simulink model "sm_import_stewart_platform"  (R2021b)
settings: Solver=ode45  StartTime=0.0  StopTime=10.0  RelTol=1e-3  EnableMultiTasking=on
model workspace (MATLAB code in the model file):
  | % The six origin vectors correspond to the six legs of the Stewart platform
  | stewart_pos_base = [0.0962 0 -0.0336; 0.0772 0 -0.0665;-0.0742 0 -0.0599;...
  |     -0.0962 0 -0.0336; -0.0190 0 0.1001;0.019 0 0.1001];
  | 
  | % Corresponding body points on the top plate
  | stewart_body_pts = [0.0607 0 0.0203; 0.0128 0 -0.0628; -0.0145 0 -0.0669; ...
  |     -0.0652 0 0.0208; -0.0507 0 0.046; 0.0507 0 0.046]';
  | 
  | % Leg length
  | leg_length = 0.19*ones(1,6);
undefined symbols (not defined in the file): X, Y, Z
libraries: sm_lib x1374, nesl_utility x19
(part 17 of 28)

== system sm_import_stewart_platform/Stewart Platform/Imported Stewart Platform/ActuatorAssm1_2/DrivenAssm_1_RIGID/CeramicStrip5010_2_RIGID ==
  ReferenceFrame : sm_lib/Frames and Transforms/Reference Frame
  Solid : sm_lib/Body Elements/File Solid  ExtGeomFileName=CeramicStrip5010_Default_sldprt.STL  UnitType=Custom  ExtGeomFileUnits=cm  StepReaderType=HEX  ExportConvexHullGeometry=off  InertiaType=Custom  Mass=0.0012937499999999978  MassUnits=kg  CenterOfMass=[-0.47402595951185544 0.93613171356507663 0]  CenterOfMassUnits=cm  MomentsOfInertia=[0.006066878906249993 0.0061722656249999933 0.00011023828124999996]  MomentsOfInertiaUnits=kg*cm^2  ProductsOfInertia=[0 0 0]  ProductsOfInertiaUnits=kg*cm^2  BasedOnType=Density  Density=1000  DensityUnits=kg/(m^3)  DoExposeReferenceFrame=on  SerializedFrames=<Frames/>  GraphicType=FromGeometry  MarkerShape=Sphere  MarkerSize=10  MarkerSizeUnits=m  GraphicVisPropType=SimpleVisualProperties  GraphicDiffuseColor=[0.95999999999999996 0.95999999999999996 0.95999999999999996]  GraphicSpecularColor=[0.5 0.5 0.5 1.0]  GraphicAmbientColor=[0.15 0.15 0.15 1.0]  GraphicEmissiveColor=[0.0 0.0 0.0 1.0]  GraphicShininess=75  GraphicOpacity=1
  F : PMIOPort  Side=Left
  connections:
  ReferenceFrame/RConn1 -- Solid/RConn1 -- F/RConn1

== system sm_import_stewart_platform/Stewart Platform/Imported Stewart Platform/ActuatorAssm1_2/DrivenAssm_1_RIGID/GratingStrip5010_1_RIGID ==
  ReferenceFrame : sm_lib/Frames and Transforms/Reference Frame
  Solid : sm_lib/Body Elements/File Solid  ExtGeomFileName=GratingStrip5010_Default_sldprt.STL  UnitType=Custom  ExtGeomFileUnits=cm  StepReaderType=HEX  ExportConvexHullGeometry=off  InertiaType=Custom  Mass=0.00056172468299999889  MassUnits=kg  CenterOfMass=[-0.84754852632874456 1.2395216473722859 3.0000000000000004]  CenterOfMassUnits=cm  MomentsOfInertia=[0.001685186808580852 0.0017040491686085529 1.8887879189411595e-05]  MomentsOfInertiaUnits=kg*cm^2  ProductsOfInertia=[0 0 0]  ProductsOfInertiaUnits=kg*cm^2  BasedOnType=Density  Density=1000  DensityUnits=kg/(m^3)  DoExposeReferenceFrame=on  SerializedFrames=<Frames/>  GraphicType=FromGeometry  MarkerShape=Sphere  MarkerSize=10  MarkerSizeUnits=m  GraphicVisPropType=SimpleVisualProperties  GraphicDiffuseColor=[0.71905882352941175 0.57976470588235285 0.21835294117647058]  GraphicSpecularColor=[0.5 0.5 0.5 1.0]  GraphicAmbientColor=[0.15 0.15 0.15 1.0]  GraphicEmissiveColor=[0.0 0.0 0.0 1.0]  GraphicShininess=75  GraphicOpacity=1
  F : PMIOPort  Side=Left
  connections:
  ReferenceFrame/RConn1 -- Solid/RConn1 -- F/RConn1

== system sm_import_stewart_platform/Stewart Platform/Imported Stewart Platform/ActuatorAssm1_2/DrivenAssm_1_RIGID/Recessed_Pan_Head_Screw_M2x8_48_Z_10_RIGID ==
  ReferenceFrame : sm_lib/Frames and Transforms/Reference Frame
  Solid : sm_lib/Body Elements/File Solid  ExtGeomFileName=Recessed_Pan_Head_Screw_M2x8_48_Z_Default_sldprt.STL  UnitType=Custom  ExtGeomFileUnits=cm  StepReaderType=HEX  ExportConvexHullGeometry=off  InertiaType=Custom  Mass=0.00030420054001085506  MassUnits=kg  CenterOfMass=[0.23057963245570592 -4.2158298307861626e-10 -1.6472469656016965e-11]  CenterOfMassUnits=cm  MomentsOfInertia=[3.0541038740142581e-06 2.6916548970402947e-05 2.6916548962268568e-05]  MomentsOfInertiaUnits=kg*cm^2  ProductsOfInertia=[0 0 0]  ProductsOfInertiaUnits=kg*cm^2  BasedOnType=Density  Density=1000  DensityUnits=kg/(m^3)  DoExposeReferenceFrame=on  SerializedFrames=<Frames/>  GraphicType=FromGeometry  MarkerShape=Sphere  MarkerSize=10  MarkerSizeUnits=m  GraphicVisPropType=SimpleVisualProperties  GraphicDiffuseColor=[0.72282352941176464 0.72282352941176464 0.72282352941176464]  GraphicSpecularColor=[0.5 0.5 0.5 1.0]  GraphicAmbientColor=[0.15 0.15 0.15 1.0]  GraphicEmissiveColor=[0.0 0.0 0.0 1.0]  GraphicShininess=75  GraphicOpacity=1
  F : PMIOPort  Side=Left
  connections:
  ReferenceFrame/RConn1 -- Solid/RConn1 -- F/RConn1

== system sm_import_stewart_platform/Stewart Platform/Imported Stewart Platform/ActuatorAssm1_2/DrivenAssm_1_RIGID/Recessed_Pan_Head_Screw_M2x8_48_Z_1_RIGID ==
  ReferenceFrame : sm_lib/Frames and Transforms/Reference Frame
  Solid : sm_lib/Body Elements/File Solid  ExtGeomFileName=Recessed_Pan_Head_Screw_M2x8_48_Z_Default_sldprt.STL  UnitType=Custom  ExtGeomFileUnits=cm  StepReaderType=HEX  ExportConvexHullGeometry=off  InertiaType=Custom  Mass=0.00030420054001085506  MassUnits=kg  CenterOfMass=[0.23057963245570592 -4.2158298307861626e-10 -1.6472469656016965e-11]  CenterOfMassUnits=cm  MomentsOfInertia=[3.0541038740142581e-06 2.6916548970402947e-05 2.6916548962268568e-05]  MomentsOfInertiaUnits=kg*cm^2  ProductsOfInertia=[0 0 0]  ProductsOfInertiaUnits=kg*cm^2  BasedOnType=Density  Density=1000  DensityUnits=kg/(m^3)  DoExposeReferenceFrame=on  SerializedFrames=<Frames/>  GraphicType=FromGeometry  MarkerShape=Sphere  MarkerSize=10  MarkerSizeUnits=m  GraphicVisPropType=SimpleVisualProperties  GraphicDiffuseColor=[0.72282352941176464 0.72282352941176464 0.72282352941176464]  GraphicSpecularColor=[0.5 0.5 0.5 1.0]  GraphicAmbientColor=[0.15 0.15 0.15 1.0]  GraphicEmissiveColor=[0.0 0.0 0.0 1.0]  GraphicShininess=75  GraphicOpacity=1
  F : PMIOPort  Side=Left
  connections:
  ReferenceFrame/RConn1 -- Solid/RConn1 -- F/RConn1

== system sm_import_stewart_platform/Stewart Platform/Imported Stewart Platform/ActuatorAssm1_2/DrivenAssm_1_RIGID/Recessed_Pan_Head_Screw_M2x8_48_Z_2_RIGID ==
  ReferenceFrame : sm_lib/Frames and Transforms/Reference Frame
  Solid : sm_lib/Body Elements/File Solid  ExtGeomFileName=Recessed_Pan_Head_Screw_M2x8_48_Z_Default_sldprt.STL  UnitType=Custom  ExtGeomFileUnits=cm  StepReaderType=HEX  ExportConvexHullGeometry=off  InertiaType=Custom  Mass=0.00030420054001085506  MassUnits=kg  CenterOfMass=[0.23057963245570592 -4.2158298307861626e-10 -1.6472469656016965e-11]  CenterOfMassUnits=cm  MomentsOfInertia=[3.0541038740142581e-06 2.6916548970402947e-05 2.6916548962268568e-05]  MomentsOfInertiaUnits=kg*cm^2  ProductsOfInertia=[0 0 0]  ProductsOfInertiaUnits=kg*cm^2  BasedOnType=Density  Density=1000  DensityUnits=kg/(m^3)  DoExposeReferenceFrame=on  SerializedFrames=<Frames/>  GraphicType=FromGeometry  MarkerShape=Sphere  MarkerSize=10  MarkerSizeUnits=m  GraphicVisPropType=SimpleVisualProperties  GraphicDiffuseColor=[0.72282352941176464 0.72282352941176464 0.72282352941176464]  GraphicSpecularColor=[0.5 0.5 0.5 1.0]  GraphicAmbientColor=[0.15 0.15 0.15 1.0]  GraphicEmissiveColor=[0.0 0.0 0.0 1.0]  GraphicShininess=75  GraphicOpacity=1
  F : PMIOPort  Side=Left
  connections:
  ReferenceFrame/RConn1 -- Solid/RConn1 -- F/RConn1

== system sm_import_stewart_platform/Stewart Platform/Imported Stewart Platform/ActuatorAssm1_2/DrivenAssm_1_RIGID/Recessed_Pan_Head_Screw_M2x8_48_Z_3_RIGID ==
  ReferenceFrame : sm_lib/Frames and Transforms/Reference Frame
  Solid : sm_lib/Body Elements/File Solid  ExtGeomFileName=Recessed_Pan_Head_Screw_M2x8_48_Z_Default_sldprt.STL  UnitType=Custom  ExtGeomFileUnits=cm  StepReaderType=HEX  ExportConvexHullGeometry=off  InertiaType=Custom  Mass=0.00030420054001085506  MassUnits=kg  CenterOfMass=[0.23057963245570592 -4.2158298307861626e-10 -1.6472469656016965e-11]  CenterOfMassUnits=cm  MomentsOfInertia=[3.0541038740142581e-06 2.6916548970402947e-05 2.6916548962268568e-05]  MomentsOfInertiaUnits=kg*cm^2  ProductsOfInertia=[0 0 0]  ProductsOfInertiaUnits=kg*cm^2  BasedOnType=Density  Density=1000  DensityUnits=kg/(m^3)  DoExposeReferenceFrame=on  SerializedFrames=<Frames/>  GraphicType=FromGeometry  MarkerShape=Sphere  MarkerSize=10  MarkerSizeUnits=m  GraphicVisPropType=SimpleVisualProperties  GraphicDiffuseColor=[0.72282352941176464 0.72282352941176464 0.72282352941176464]  GraphicSpecularColor=[0.5 0.5 0.5 1.0]  GraphicAmbientColor=[0.15 0.15 0.15 1.0]  GraphicEmissiveColor=[0.0 0.0 0.0 1.0]  GraphicShininess=75  GraphicOpacity=1
  F : PMIOPort  Side=Left
  connections:
  ReferenceFrame/RConn1 -- Solid/RConn1 -- F/RConn1

== system sm_import_stewart_platform/Stewart Platform/Imported Stewart Platform/ActuatorAssm1_2/DrivenAssm_1_RIGID/Recessed_Pan_Head_Screw_M2x8_48_Z_4_RIGID ==
  ReferenceFrame : sm_lib/Frames and Transforms/Reference Frame
  Solid : sm_lib/Body Elements/File Solid  ExtGeomFileName=Recessed_Pan_Head_Screw_M2x8_48_Z_Default_sldprt.STL  UnitType=Custom  ExtGeomFileUnits=cm  StepReaderType=HEX  ExportConvexHullGeometry=off  InertiaType=Custom  Mass=0.00030420054001085506  MassUnits=kg  CenterOfMass=[0.23057963245570592 -4.2158298307861626e-10 -1.6472469656016965e-11]  CenterOfMassUnits=cm  MomentsOfInertia=[3.0541038740142581e-06 2.6916548970402947e-05 2.6916548962268568e-05]  MomentsOfInertiaUnits=kg*cm^2  ProductsOfInertia=[0 0 0]  ProductsOfInertiaUnits=kg*cm^2  BasedOnType=Density  Density=1000  DensityUnits=kg/(m^3)  DoExposeReferenceFrame=on  SerializedFrames=<Frames/>  GraphicType=FromGeometry  MarkerShape=Sphere  MarkerSize=10  MarkerSizeUnits=m  GraphicVisPropType=SimpleVisualProperties  GraphicDiffuseColor=[0.72282352941176464 0.72282352941176464 0.72282352941176464]  GraphicSpecularColor=[0.5 0.5 0.5 1.0]  GraphicAmbientColor=[0.15 0.15 0.15 1.0]  GraphicEmissiveColor=[0.0 0.0 0.0 1.0]  GraphicShininess=75  GraphicOpacity=1
  F : PMIOPort  Side=Left
  connections:
  ReferenceFrame/RConn1 -- Solid/RConn1 -- F/RConn1

== system sm_import_stewart_platform/Stewart Platform/Imported Stewart Platform/ActuatorAssm1_2/DrivenAssm_1_RIGID/Recessed_Pan_Head_Screw_M2x8_48_Z_5_RIGID ==
  ReferenceFrame : sm_lib/Frames and Transforms/Reference Frame
  Solid : sm_lib/Body Elements/File Solid  ExtGeomFileName=Recessed_Pan_Head_Screw_M2x8_48_Z_Default_sldprt.STL  UnitType=Custom  ExtGeomFileUnits=cm  StepReaderType=HEX  ExportConvexHullGeometry=off  InertiaType=Custom  Mass=0.00030420054001085506  MassUnits=kg  CenterOfMass=[0.23057963245570592 -4.2158298307861626e-10 -1.6472469656016965e-11]  CenterOfMassUnits=cm  MomentsOfInertia=[3.0541038740142581e-06 2.6916548970402947e-05 2.6916548962268568e-05]  MomentsOfInertiaUnits=kg*cm^2  ProductsOfInertia=[0 0 0]  ProductsOfInertiaUnits=kg*cm^2  BasedOnType=Density  Density=1000  DensityUnits=kg/(m^3)  DoExposeReferenceFrame=on  SerializedFrames=<Frames/>  GraphicType=FromGeometry  MarkerShape=Sphere  MarkerSize=10  MarkerSizeUnits=m  GraphicVisPropType=SimpleVisualProperties  GraphicDiffuseColor=[0.72282352941176464 0.72282352941176464 0.72282352941176464]  GraphicSpecularColor=[0.5 0.5 0.5 1.0]  GraphicAmbientColor=[0.15 0.15 0.15 1.0]  GraphicEmissiveColor=[0.0 0.0 0.0 1.0]  GraphicShininess=75  GraphicOpacity=1
  F : PMIOPort  Side=Left
  connections:
  ReferenceFrame/RConn1 -- Solid/RConn1 -- F/RConn1

== system sm_import_stewart_platform/Stewart Platform/Imported Stewart Platform/ActuatorAssm1_2/DrivenAssm_1_RIGID/Recessed_Pan_Head_Screw_M2x8_48_Z_6_RIGID ==
  ReferenceFrame : sm_lib/Frames and Transforms/Reference Frame
  Solid : sm_lib/Body Elements/File Solid  ExtGeomFileName=Recessed_Pan_Head_Screw_M2x8_48_Z_Default_sldprt.STL  UnitType=Custom  ExtGeomFileUnits=cm  StepReaderType=HEX  ExportConvexHullGeometry=off  InertiaType=Custom  Mass=0.00030420054001085506  MassUnits=kg  CenterOfMass=[0.23057963245570592 -4.2158298307861626e-10 -1.6472469656016965e-11]  CenterOfMassUnits=cm  MomentsOfInertia=[3.0541038740142581e-06 2.6916548970402947e-05 2.6916548962268568e-05]  MomentsOfInertiaUnits=kg*cm^2  ProductsOfInertia=[0 0 0]  ProductsOfInertiaUnits=kg*cm^2  BasedOnType=Density  Density=1000  DensityUnits=kg/(m^3)  DoExposeReferenceFrame=on  SerializedFrames=<Frames/>  GraphicType=FromGeometry  MarkerShape=Sphere  MarkerSize=10  MarkerSizeUnits=m  GraphicVisPropType=SimpleVisualProperties  GraphicDiffuseColor=[0.72282352941176464 0.72282352941176464 0.72282352941176464]  GraphicSpecularColor=[0.5 0.5 0.5 1.0]  GraphicAmbientColor=[0.15 0.15 0.15 1.0]  GraphicEmissiveColor=[0.0 0.0 0.0 1.0]  GraphicShininess=75  GraphicOpacity=1
  F : PMIOPort  Side=Left
  connections:
  ReferenceFrame/RConn1 -- Solid/RConn1 -- F/RConn1

== system sm_import_stewart_platform/Stewart Platform/Imported Stewart Platform/ActuatorAssm1_2/DrivenAssm_1_RIGID/Recessed_Pan_Head_Screw_M2x8_48_Z_7_RIGID ==
  ReferenceFrame : sm_lib/Frames and Transforms/Reference Frame
  Solid : sm_lib/Body Elements/File Solid  ExtGeomFileName=Recessed_Pan_Head_Screw_M2x8_48_Z_Default_sldprt.STL  UnitType=Custom  ExtGeomFileUnits=cm  StepReaderType=HEX  ExportConvexHullGeometry=off  InertiaType=Custom  Mass=0.00030420054001085506  MassUnits=kg  CenterOfMass=[0.23057963245570592 -4.2158298307861626e-10 -1.6472469656016965e-11]  CenterOfMassUnits=cm  MomentsOfInertia=[3.0541038740142581e-06 2.6916548970402947e-05 2.6916548962268568e-05]  MomentsOfInertiaUnits=kg*cm^2  ProductsOfInertia=[0 0 0]  ProductsOfInertiaUnits=kg*cm^2  BasedOnType=Density  Density=1000  DensityUnits=kg/(m^3)  DoExposeReferenceFrame=on  SerializedFrames=<Frames/>  GraphicType=FromGeometry  MarkerShape=Sphere  MarkerSize=10  MarkerSizeUnits=m  GraphicVisPropType=SimpleVisualProperties  GraphicDiffuseColor=[0.72282352941176464 0.72282352941176464 0.72282352941176464]  GraphicSpecularColor=[0.5 0.5 0.5 1.0]  GraphicAmbientColor=[0.15 0.15 0.15 1.0]  GraphicEmissiveColor=[0.0 0.0 0.0 1.0]  GraphicShininess=75  GraphicOpacity=1
  F : PMIOPort  Side=Left
  connections:
  ReferenceFrame/RConn1 -- Solid/RConn1 -- F/RConn1

== system sm_import_stewart_platform/Stewart Platform/Imported Stewart Platform/ActuatorAssm1_2/DrivenAssm_1_RIGID/Recessed_Pan_Head_Screw_M2x8_48_Z_8_RIGID ==
  ReferenceFrame : sm_lib/Frames and Transforms/Reference Frame
  Solid : sm_lib/Body Elements/File Solid  ExtGeomFileName=Recessed_Pan_Head_Screw_M2x8_48_Z_Default_sldprt.STL  UnitType=Custom  ExtGeomFileUnits=cm  StepReaderType=HEX  ExportConvexHullGeometry=off  InertiaType=Custom  Mass=0.00030420054001085506  MassUnits=kg  CenterOfMass=[0.23057963245570592 -4.2158298307861626e-10 -1.6472469656016965e-11]  CenterOfMassUnits=cm  MomentsOfInertia=[3.0541038740142581e-06 2.6916548970402947e-05 2.6916548962268568e-05]  MomentsOfInertiaUnits=kg*cm^2  ProductsOfInertia=[0 0 0]  ProductsOfInertiaUnits=kg*cm^2  BasedOnType=Density  Density=1000  DensityUnits=kg/(m^3)  DoExposeReferenceFrame=on  SerializedFrames=<Frames/>  GraphicType=FromGeometry  MarkerShape=Sphere  MarkerSize=10  MarkerSizeUnits=m  GraphicVisPropType=SimpleVisualProperties  GraphicDiffuseColor=[0.72282352941176464 0.72282352941176464 0.72282352941176464]  GraphicSpecularColor=[0.5 0.5 0.5 1.0]  GraphicAmbientColor=[0.15 0.15 0.15 1.0]  GraphicEmissiveColor=[0.0 0.0 0.0 1.0]  GraphicShininess=75  GraphicOpacity=1
  F : PMIOPort  Side=Left
  connections:
  ReferenceFrame/RConn1 -- Solid/RConn1 -- F/RConn1

== system sm_import_stewart_platform/Stewart Platform/Imported Stewart Platform/ActuatorAssm1_2/DrivenAssm_1_RIGID/Recessed_Pan_Head_Screw_M2x8_48_Z_9_RIGID ==
  ReferenceFrame : sm_lib/Frames and Transforms/Reference Frame
  Solid : sm_lib/Body Elements/File Solid  ExtGeomFileName=Recessed_Pan_Head_Screw_M2x8_48_Z_Default_sldprt.STL  UnitType=Custom  ExtGeomFileUnits=cm  StepReaderType=HEX  ExportConvexHullGeometry=off  InertiaType=Custom  Mass=0.00030420054001085506  MassUnits=kg  CenterOfMass=[0.23057963245570592 -4.2158298307861626e-10 -1.6472469656016965e-11]  CenterOfMassUnits=cm  MomentsOfInertia=[3.0541038740142581e-06 2.6916548970402947e-05 2.6916548962268568e-05]  MomentsOfInertiaUnits=kg*cm^2  ProductsOfInertia=[0 0 0]  ProductsOfInertiaUnits=kg*cm^2  BasedOnType=Density  Density=1000  DensityUnits=kg/(m^3)  DoExposeReferenceFrame=on  SerializedFrames=<Frames/>  GraphicType=FromGeometry  MarkerShape=Sphere  MarkerSize=10  MarkerSizeUnits=m  GraphicVisPropType=SimpleVisualProperties  GraphicDiffuseColor=[0.72282352941176464 0.72282352941176464 0.72282352941176464]  GraphicSpecularColor=[0.5 0.5 0.5 1.0]  GraphicAmbientColor=[0.15 0.15 0.15 1.0]  GraphicEmissiveColor=[0.0 0.0 0.0 1.0]  GraphicShininess=75  GraphicOpacity=1
  F : PMIOPort  Side=Left
  connections:
  ReferenceFrame/RConn1 -- Solid/RConn1 -- F/RConn1

== system sm_import_stewart_platform/Stewart Platform/Imported Stewart Platform/ActuatorAssm1_2/DrivenAssm_1_RIGID/SV2075_1_RIGID ==
  ReferenceFrame : sm_lib/Frames and Transforms/Reference Frame
  Solid : sm_lib/Body Elements/File Solid  ExtGeomFileName=SV2075_Default_sldprt.STL  UnitType=Custom  ExtGeomFileUnits=cm  StepReaderType=HEX  ExportConvexHullGeometry=off  InertiaType=Custom  Mass=0.0058459106101348196  MassUnits=kg  CenterOfMass=[-0.3298949175327261 0.0096923486215533452 3.75]  CenterOfMassUnits=cm  MomentsOfInertia=[0.027698839272727555 0.027673933267832958 0.00032822959311509738]  MomentsOfInertiaUnits=kg*cm^2  ProductsOfInertia=[0 0 1.1416492577499715e-06]  ProductsOfInertiaUnits=kg*cm^2  BasedOnType=Density  Density=1000  DensityUnits=kg/(m^3)  DoExposeReferenceFrame=on  SerializedFrames=<Frames/>  GraphicType=FromGeometry  MarkerShape=Sphere  MarkerSize=10  MarkerSizeUnits=m  GraphicVisPropType=SimpleVisualProperties  GraphicDiffuseColor=[0.97999999999999998 0.97999999999999998 0.97999999999999998]  GraphicSpecularColor=[0.5 0.5 0.5 1.0]  GraphicAmbientColor=[0.15 0.15 0.15 1.0]  GraphicEmissiveColor=[0.0 0.0 0.0 1.0]  GraphicShininess=75  GraphicOpacity=1
  F : PMIOPort  Side=Left
  connections:
  ReferenceFrame/RConn1 -- Solid/RConn1 -- F/RConn1

== system sm_import_stewart_platform/Stewart Platform/Imported Stewart Platform/ActuatorAssm1_2/DrivenAssm_1_RIGID/SV2075_2_RIGID ==
  ReferenceFrame : sm_lib/Frames and Transforms/Reference Frame
  Solid : sm_lib/Body Elements/File Solid  ExtGeomFileName=SV2075_Default_sldprt.STL  UnitType=Custom  ExtGeomFileUnits=cm  StepReaderType=HEX  ExportConvexHullGeometry=off  InertiaType=Custom  Mass=0.0058459106101348196  MassUnits=kg  CenterOfMass=[-0.3298949175327261 0.0096923486215533452 3.75]  CenterOfMassUnits=cm  MomentsOfInertia=[0.027698839272727555 0.027673933267832958 0.00032822959311509738]  MomentsOfInertiaUnits=kg*cm^2  ProductsOfInertia=[0 0 1.1416492577499715e-06]  ProductsOfInertiaUnits=kg*cm^2  BasedOnType=Density  Density=1000  DensityUnits=kg/(m^3)  DoExposeReferenceFrame=on  SerializedFrames=<Frames/>  GraphicType=FromGeometry  MarkerShape=Sphere  MarkerSize=10  MarkerSizeUnits=m  GraphicVisPropType=SimpleVisualProperties  GraphicDiffuseColor=[0.97999999999999998 0.97999999999999998 0.97999999999999998]  GraphicSpecularColor=[0.5 0.5 0.5 1.0]  GraphicAmbientColor=[0.15 0.15 0.15 1.0]  GraphicEmissiveColor=[0.0 0.0 0.0 1.0]  GraphicShininess=75  GraphicOpacity=1
  F : PMIOPort  Side=Left
  connections:
  ReferenceFrame/RConn1 -- Solid/RConn1 -- F/RConn1

== system sm_import_stewart_platform/Stewart Platform/Imported Stewart Platform/ActuatorAssm1_2/DrivenAssm_1_RIGID/Yoke_1_RIGID ==
  ReferenceFrame : sm_lib/Frames and Transforms/Reference Frame
  Solid : sm_lib/Body Elements/File Solid  ExtGeomFileName=Yoke_Default_sldprt.STL  UnitType=Custom  ExtGeomFileUnits=m  StepReaderType=HEX  ExportConvexHullGeometry=off  InertiaType=Custom  Mass=0.0085668068985893069  MassUnits=kg  CenterOfMass=[3.3036113322449594e-09 4.5392080360257641e-09 0.013809135161090778]  CenterOfMassUnits=m  MomentsOfInertia=[3.6198630707133227e-07 3.7260728672028368e-07 1.1777278033424778e-07]  MomentsOfInertiaUnits=kg*m^2  ProductsOfInertia=[1.5891854780888145e-13 3.9281797530062808e-13 -1.9646780999777998e-13]  ProductsOfInertiaUnits=kg*m^2  BasedOnType=Density  Density=1000  DensityUnits=kg/(m^3)  DoExposeReferenceFrame=on  SerializedFrames=<Frames/>  GraphicType=FromGeometry  MarkerShape=Sphere  MarkerSize=10  MarkerSizeUnits=m  GraphicVisPropType=SimpleVisualProperties  GraphicDiffuseColor=[0.77647058823529413 0.75686274509803919 0.73725490196078436]  GraphicSpecularColor=[0.5 0.5 0.5 1.0]  GraphicAmbientColor=[0.15 0.15 0.15 1.0]  GraphicEmissiveColor=[0.0 0.0 0.0 1.0]  GraphicShininess=75  GraphicOpacity=1
  F : PMIOPort  Side=Left
  connections:
  ReferenceFrame/RConn1 -- Solid/RConn1 -- F/RConn1

== system sm_import_stewart_platform/Stewart Platform/Imported Stewart Platform/ActuatorAssm1_2/DrivenAssm_1_RIGID/pin2_1_RIGID ==
  ReferenceFrame : sm_lib/Frames and Transforms/Reference Frame
  Solid : sm_lib/Body Elements/File Solid  ExtGeomFileName=pin2_Default_sldprt.STL  UnitType=Custom  ExtGeomFileUnits=cm  StepReaderType=HEX  ExportConvexHullGeometry=off  InertiaType=Custom  Mass=0.0030640524011317904  MassUnits=kg  CenterOfMass=[0.62878050766606708 1.2281931362555856e-05 9.2878917417835236e-08]  CenterOfMassUnits=cm  MomentsOfInertia=[0.00015143303511498066 0.00047164024915314555 0.00047162614442519934]  MomentsOfInertiaUnits=kg*cm^2  ProductsOfInertia=[-9.4727819805528836e-10 1.4280711810645117e-10 1.8883664164919476e-08]  ProductsOfInertiaUnits=kg*cm^2  BasedOnType=Density  Density=1000  DensityUnits=kg/(m^3)  DoExposeReferenceFrame=on  SerializedFrames=<Frames/>  GraphicType=FromGeometry  MarkerShape=Sphere  MarkerSize=10  MarkerSizeUnits=m  GraphicVisPropType=SimpleVisualProperties  GraphicDiffuseColor=[0.72282352941176464 0.72282352941176464 0.72282352941176464]  GraphicSpecularColor=[0.5 0.5 0.5 1.0]  GraphicAmbientColor=[0.15 0.15 0.15 1.0]  GraphicEmissiveColor=[0.0 0.0 0.0 1.0]  GraphicShininess=75  GraphicOpacity=1
  F : PMIOPort  Side=Left
  connections:
  ReferenceFrame/RConn1 -- Solid/RConn1 -- F/RConn1

== system sm_import_stewart_platform/Stewart Platform/Imported Stewart Platform/ActuatorAssm2_2/CarrierAssm_1_RIGID/Carrier_Block_1_RIGID ==
  ReferenceFrame : sm_lib/Frames and Transforms/Reference Frame
  Solid : sm_lib/Body Elements/File Solid  ExtGeomFileName=Carrier_Block_Default_sldprt.STL  UnitType=Custom  ExtGeomFileUnits=m  StepReaderType=HEX  ExportConvexHullGeometry=off  InertiaType=Custom  Mass=0.29755503214781071  MassUnits=kg  CenterOfMass=[0.052371592454755117 -0.00023155972844887416 0.0090326123177344834]  CenterOfMassUnits=m  MomentsOfInertia=[0.00011632507036741897 0.00038061460758238494 0.00046776142289895373]  MomentsOfInertiaUnits=kg*m^2  ProductsOfInertia=[-7.7054025601460358e-07 -8.2627224851298449e-06 -5.2656093991147314e-07]  ProductsOfInertiaUnits=kg*m^2  BasedOnType=Density  Density=1000  DensityUnits=kg/(m^3)  DoExposeReferenceFrame=on  SerializedFrames=<Frames/>  GraphicType=FromGeometry  MarkerShape=Sphere  MarkerSize=10  MarkerSizeUnits=m  GraphicVisPropType=SimpleVisualProperties  GraphicDiffuseColor=[0.21568627450980393 0.60784313725490191 1]  GraphicSpecularColor=[0.5 0.5 0.5 1.0]  GraphicAmbientColor=[0.15 0.15 0.15 1.0]  GraphicEmissiveColor=[0.0 0.0 0.0 1.0]  GraphicShininess=75  GraphicOpacity=1
  F : PMIOPort  Side=Left
  connections:
  ReferenceFrame/RConn1 -- Solid/RConn1 -- F/RConn1

== system sm_import_stewart_platform/Stewart Platform/Imported Stewart Platform/ActuatorAssm2_2/CarrierAssm_1_RIGID/Cylinder_Head_Cap_Screw_M3x8_1_RIGID ==
  ReferenceFrame : sm_lib/Frames and Transforms/Reference Frame
  Solid : sm_lib/Body Elements/File Solid  ExtGeomFileName=Cylinder_Head_Cap_Screw_M3x8_Default_sldprt.STL  UnitType=Custom  ExtGeomFileUnits=cm  StepReaderType=HEX  ExportConvexHullGeometry=off  InertiaType=Custom  Mass=0.00075681554585630491  MassUnits=kg  CenterOfMass=[0.18814854043794096 4.2404888903707961e-05 3.0314199022387744e-07]  CenterOfMassUnits=cm  MomentsOfInertia=[1.8441866345461375e-05 7.8616006686727758e-05 7.8603749633107087e-05]  MomentsOfInertiaUnits=kg*cm^2  ProductsOfInertia=[-8.295565631821646e-10 6.6108014175054549e-11 9.2474917315283758e-09]  ProductsOfInertiaUnits=kg*cm^2  BasedOnType=Density  Density=1000  DensityUnits=kg/(m^3)  DoExposeReferenceFrame=on  SerializedFrames=<Frames/>  GraphicType=FromGeometry  MarkerShape=Sphere  MarkerSize=10  MarkerSizeUnits=m  GraphicVisPropType=SimpleVisualProperties  GraphicDiffuseColor=[0.72282352941176464 0.72282352941176464 0.72282352941176464]  GraphicSpecularColor=[0.5 0.5 0.5 1.0]  GraphicAmbientColor=[0.15 0.15 0.15 1.0]  GraphicEmissiveColor=[0.0 0.0 0.0 1.0]  GraphicShininess=75  GraphicOpacity=1
  F : PMIOPort  Side=Left
  connections:
  ReferenceFrame/RConn1 -- Solid/RConn1 -- F/RConn1

== system sm_import_stewart_platform/Stewart Platform/Imported Stewart Platform/ActuatorAssm2_2/CarrierAssm_1_RIGID/Cylinder_Head_Cap_Screw_M3x8_2_RIGID ==
  ReferenceFrame : sm_lib/Frames and Transforms/Reference Frame
  Solid : sm_lib/Body Elements/File Solid  ExtGeomFileName=Cylinder_Head_Cap_Screw_M3x8_Default_sldprt.STL  UnitType=Custom  ExtGeomFileUnits=cm  StepReaderType=HEX  ExportConvexHullGeometry=off  InertiaType=Custom  Mass=0.00075681554585630491  MassUnits=kg  CenterOfMass=[0.18814854043794096 4.2404888903707961e-05 3.0314199022387744e-07]  CenterOfMassUnits=cm  MomentsOfInertia=[1.8441866345461375e-05 7.8616006686727758e-05 7.8603749633107087e-05]  MomentsOfInertiaUnits=kg*cm^2  ProductsOfInertia=[-8.295565631821646e-10 6.6108014175054549e-11 9.2474917315283758e-09]  ProductsOfInertiaUnits=kg*cm^2  BasedOnType=Density  Density=1000  DensityUnits=kg/(m^3)  DoExposeReferenceFrame=on  SerializedFrames=<Frames/>  GraphicType=FromGeometry  MarkerShape=Sphere  MarkerSize=10  MarkerSizeUnits=m  GraphicVisPropType=SimpleVisualProperties  GraphicDiffuseColor=[0.72282352941176464 0.72282352941176464 0.72282352941176464]  GraphicSpecularColor=[0.5 0.5 0.5 1.0]  GraphicAmbientColor=[0.15 0.15 0.15 1.0]  GraphicEmissiveColor=[0.0 0.0 0.0 1.0]  GraphicShininess=75  GraphicOpacity=1
  F : PMIOPort  Side=Left
  connections:
  ReferenceFrame/RConn1 -- Solid/RConn1 -- F/RConn1

== system sm_import_stewart_platform/Stewart Platform/Imported Stewart Platform/ActuatorAssm2_2/CarrierAssm_1_RIGID/HR_1_Motor_1_RIGID ==
  ReferenceFrame : sm_lib/Frames and Transforms/Reference Frame
  Solid : sm_lib/Body Elements/File Solid  ExtGeomFileName=HR_1_Motor_Default_sldprt.STL  UnitType=Custom  ExtGeomFileUnits=cm  StepReaderType=HEX  ExportConvexHullGeometry=off  InertiaType=Custom  Mass=0.016323277951690116  MassUnits=kg  CenterOfMass=[1.1461762495150611 1.9087990143138187 0.39999826480475109]  CenterOfMassUnits=cm  MomentsOfInertia=[0.022976248526302246 0.016967187564536409 0.038272540312041692]  MomentsOfInertiaUnits=kg*cm^2  ProductsOfInertia=[-6.3449814973716521e-08 -1.4415405966206584e-07 -0.0031628803180496112]  ProductsOfInertiaUnits=kg*cm^2  BasedOnType=Density  Density=1000  DensityUnits=kg/(m^3)  DoExposeReferenceFrame=on  SerializedFrames=<Frames/>  GraphicType=FromGeometry  MarkerShape=Sphere  MarkerSize=10  MarkerSizeUnits=m  GraphicVisPropType=SimpleVisualProperties  GraphicDiffuseColor=[0.95999999999999996 0.69647058823529406 0.56847058823529406]  GraphicSpecularColor=[0.5 0.5 0.5 1.0]  GraphicAmbientColor=[0.15 0.15 0.15 1.0]  GraphicEmissiveColor=[0.0 0.0 0.0 1.0]  GraphicShininess=75  GraphicOpacity=1
  F : PMIOPort  Side=Left
  connections:
  ReferenceFrame/RConn1 -- Solid/RConn1 -- F/RConn1

== system sm_import_stewart_platform/Stewart Platform/Imported Stewart Platform/ActuatorAssm2_2/CarrierAssm_1_RIGID/HR_1_Motor_2_RIGID ==
  ReferenceFrame : sm_lib/Frames and Transforms/Reference Frame
  Solid : sm_lib/Body Elements/File Solid  ExtGeomFileName=HR_1_Motor_Default_sldprt.STL  UnitType=Custom  ExtGeomFileUnits=cm  StepReaderType=HEX  ExportConvexHullGeometry=off  InertiaType=Custom  Mass=0.016323277951690116  MassUnits=kg  CenterOfMass=[1.1461762495150611 1.9087990143138187 0.39999826480475109]  CenterOfMassUnits=cm  MomentsOfInertia=[0.022976248526302246 0.016967187564536409 0.038272540312041692]  MomentsOfInertiaUnits=kg*cm^2  ProductsOfInertia=[-6.3449814973716521e-08 -1.4415405966206584e-07 -0.0031628803180496112]  ProductsOfInertiaUnits=kg*cm^2  BasedOnType=Density  Density=1000  DensityUnits=kg/(m^3)  DoExposeReferenceFrame=on  SerializedFrames=<Frames/>  GraphicType=FromGeometry  MarkerShape=Sphere  MarkerSize=10  MarkerSizeUnits=m  GraphicVisPropType=SimpleVisualProperties  GraphicDiffuseColor=[0.95999999999999996 0.69647058823529406 0.56847058823529406]  GraphicSpecularColor=[0.5 0.5 0.5 1.0]  GraphicAmbientColor=[0.15 0.15 0.15 1.0]  GraphicEmissiveColor=[0.0 0.0 0.0 1.0]  GraphicShininess=75  GraphicOpacity=1
  F : PMIOPort  Side=Left
  connections:
  ReferenceFrame/RConn1 -- Solid/RConn1 -- F/RConn1

== system sm_import_stewart_platform/Stewart Platform/Imported Stewart Platform/ActuatorAssm2_2/CarrierAssm_1_RIGID/Hexagon_Socket_Button_Head_Screw_M3x6_1_RIGID ==
  ReferenceFrame : sm_lib/Frames and Transforms/Reference Frame
  Solid : sm_lib/Body Elements/File Solid  ExtGeomFileName=Hexagon_Socket_Button_Head_Screw_M3x6_Default_sldprt.STL  UnitType=Custom  ExtGeomFileUnits=cm  StepReaderType=HEX  ExportConvexHullGeometry=off  InertiaType=Custom  Mass=0.00056348185373580135  MassUnits=kg  CenterOfMass=[0.14356282026314221 8.1476592298985412e-06 5.8788316934839061e-08]  CenterOfMassUnits=cm  MomentsOfInertia=[1.3098988700385332e-05 3.5078394083955334e-05 3.5077439490752727e-05]  MomentsOfInertiaUnits=kg*cm^2  ProductsOfInertia=[-6.7519077190030419e-11 7.6873810692743504e-12 1.0654186206953444e-09]  ProductsOfInertiaUnits=kg*cm^2  BasedOnType=Density  Density=1000  DensityUnits=kg/(m^3)  DoExposeReferenceFrame=on  SerializedFrames=<Frames/>  GraphicType=FromGeometry  MarkerShape=Sphere  MarkerSize=10  MarkerSizeUnits=m  GraphicVisPropType=SimpleVisualProperties  GraphicDiffuseColor=[0.72282352941176464 0.72282352941176464 0.72282352941176464]  GraphicSpecularColor=[0.5 0.5 0.5 1.0]  GraphicAmbientColor=[0.15 0.15 0.15 1.0]  GraphicEmissiveColor=[0.0 0.0 0.0 1.0]  GraphicShininess=75  GraphicOpacity=1
  F : PMIOPort  Side=Left
  connections:
  ReferenceFrame/RConn1 -- Solid/RConn1 -- F/RConn1

== system sm_import_stewart_platform/Stewart Platform/Imported Stewart Platform/ActuatorAssm2_2/CarrierAssm_1_RIGID/Hexagon_Socket_Button_Head_Screw_M3x6_2_RIGID ==
  ReferenceFrame : sm_lib/Frames and Transforms/Reference Frame
  Solid : sm_lib/Body Elements/File Solid  ExtGeomFileName=Hexagon_Socket_Button_Head_Screw_M3x6_Default_sldprt.STL  UnitType=Custom  ExtGeomFileUnits=cm  StepReaderType=HEX  ExportConvexHullGeometry=off  InertiaType=Custom  Mass=0.00056348185373580135  MassUnits=kg  CenterOfMass=[0.14356282026314221 8.1476592298985412e-06 5.8788316934839061e-08]  CenterOfMassUnits=cm  MomentsOfInertia=[1.3098988700385332e-05 3.5078394083955334e-05 3.5077439490752727e-05]  MomentsOfInertiaUnits=kg*cm^2  ProductsOfInertia=[-6.7519077190030419e-11 7.6873810692743504e-12 1.0654186206953444e-09]  ProductsOfInertiaUnits=kg*cm^2  BasedOnType=Density  Density=1000  DensityUnits=kg/(m^3)  DoExposeReferenceFrame=on  SerializedFrames=<Frames/>  GraphicType=FromGeometry  MarkerShape=Sphere  MarkerSize=10  MarkerSizeUnits=m  GraphicVisPropType=SimpleVisualProperties  GraphicDiffuseColor=[0.72282352941176464 0.72282352941176464 0.72282352941176464]  GraphicSpecularColor=[0.5 0.5 0.5 1.0]  GraphicAmbientColor=[0.15 0.15 0.15 1.0]  GraphicEmissiveColor=[0.0 0.0 0.0 1.0]  GraphicShininess=75  GraphicOpacity=1
  F : PMIOPort  Side=Left
  connections:
  ReferenceFrame/RConn1 -- Solid/RConn1 -- F/RConn1

== system sm_import_stewart_platform/Stewart Platform/Imported Stewart Platform/ActuatorAssm2_2/CarrierAssm_1_RIGID/Hexagon_Socket_Button_Head_Screw_M3x6_3_RIGID ==
  ReferenceFrame : sm_lib/Frames and Transforms/Reference Frame
  Solid : sm_lib/Body Elements/File Solid  ExtGeomFileName=Hexagon_Socket_Button_Head_Screw_M3x6_Default_sldprt.STL  UnitType=Custom  ExtGeomFileUnits=cm  StepReaderType=HEX  ExportConvexHullGeometry=off  InertiaType=Custom  Mass=0.00056348185373580135  MassUnits=kg  CenterOfMass=[0.14356282026314221 8.1476592298985412e-06 5.8788316934839061e-08]  CenterOfMassUnits=cm  MomentsOfInertia=[1.3098988700385332e-05 3.5078394083955334e-05 3.5077439490752727e-05]  MomentsOfInertiaUnits=kg*cm^2  ProductsOfInertia=[-6.7519077190030419e-11 7.6873810692743504e-12 1.0654186206953444e-09]  ProductsOfInertiaUnits=kg*cm^2  BasedOnType=Density  Density=1000  DensityUnits=kg/(m^3)  DoExposeReferenceFrame=on  SerializedFrames=<Frames/>  GraphicType=FromGeometry  MarkerShape=Sphere  MarkerSize=10  MarkerSizeUnits=m  GraphicVisPropType=SimpleVisualProperties  GraphicDiffuseColor=[0.72282352941176464 0.72282352941176464 0.72282352941176464]  GraphicSpecularColor=[0.5 0.5 0.5 1.0]  GraphicAmbientColor=[0.15 0.15 0.15 1.0]  GraphicEmissiveColor=[0.0 0.0 0.0 1.0]  GraphicShininess=75  GraphicOpacity=1
  F : PMIOPort  Side=Left
  connections:
  ReferenceFrame/RConn1 -- Solid/RConn1 -- F/RConn1

== system sm_import_stewart_platform/Stewart Platform/Imported Stewart Platform/ActuatorAssm2_2/CarrierAssm_1_RIGID/Hexagon_Socket_Button_Head_Screw_M3x6_4_RIGID ==
  ReferenceFrame : sm_lib/Frames and Transforms/Reference Frame
  Solid : sm_lib/Body Elements/File Solid  ExtGeomFileName=Hexagon_Socket_Button_Head_Screw_M3x6_Default_sldprt.STL  UnitType=Custom  ExtGeomFileUnits=cm  StepReaderType=HEX  ExportConvexHullGeometry=off  InertiaType=Custom  Mass=0.00056348185373580135  MassUnits=kg  CenterOfMass=[0.14356282026314221 8.1476592298985412e-06 5.8788316934839061e-08]  CenterOfMassUnits=cm  MomentsOfInertia=[1.3098988700385332e-05 3.5078394083955334e-05 3.5077439490752727e-05]  MomentsOfInertiaUnits=kg*cm^2  ProductsOfInertia=[-6.7519077190030419e-11 7.6873810692743504e-12 1.0654186206953444e-09]  ProductsOfInertiaUnits=kg*cm^2  BasedOnType=Density  Density=1000  DensityUnits=kg/(m^3)  DoExposeReferenceFrame=on  SerializedFrames=<Frames/>  GraphicType=FromGeometry  MarkerShape=Sphere  MarkerSize=10  MarkerSizeUnits=m  GraphicVisPropType=SimpleVisualProperties  GraphicDiffuseColor=[0.72282352941176464 0.72282352941176464 0.72282352941176464]  GraphicSpecularColor=[0.5 0.5 0.5 1.0]  GraphicAmbientColor=[0.15 0.15 0.15 1.0]  GraphicEmissiveColor=[0.0 0.0 0.0 1.0]  GraphicShininess=75  GraphicOpacity=1
  F : PMIOPort  Side=Left
  connections:
  ReferenceFrame/RConn1 -- Solid/RConn1 -- F/RConn1

== system sm_import_stewart_platform/Stewart Platform/Imported Stewart Platform/ActuatorAssm2_2/CarrierAssm_1_RIGID/Hexagon_Socket_Button_Head_Screw_M3x6_5_RIGID ==
  ReferenceFrame : sm_lib/Frames and Transforms/Reference Frame
  Solid : sm_lib/Body Elements/File Solid  ExtGeomFileName=Hexagon_Socket_Button_Head_Screw_M3x6_Default_sldprt.STL  UnitType=Custom  ExtGeomFileUnits=cm  StepReaderType=HEX  ExportConvexHullGeometry=off  InertiaType=Custom  Mass=0.00056348185373580135  MassUnits=kg  CenterOfMass=[0.14356282026314221 8.1476592298985412e-06 5.8788316934839061e-08]  CenterOfMassUnits=cm  MomentsOfInertia=[1.3098988700385332e-05 3.5078394083955334e-05 3.5077439490752727e-05]  MomentsOfInertiaUnits=kg*cm^2  ProductsOfInertia=[-6.7519077190030419e-11 7.6873810692743504e-12 1.0654186206953444e-09]  ProductsOfInertiaUnits=kg*cm^2  BasedOnType=Density  Density=1000  DensityUnits=kg/(m^3)  DoExposeReferenceFrame=on  SerializedFrames=<Frames/>  GraphicType=FromGeometry  MarkerShape=Sphere  MarkerSize=10  MarkerSizeUnits=m  GraphicVisPropType=SimpleVisualProperties  GraphicDiffuseColor=[0.72282352941176464 0.72282352941176464 0.72282352941176464]  GraphicSpecularColor=[0.5 0.5 0.5 1.0]  GraphicAmbientColor=[0.15 0.15 0.15 1.0]  GraphicEmissiveColor=[0.0 0.0 0.0 1.0]  GraphicShininess=75  GraphicOpacity=1
  F : PMIOPort  Side=Left
  connections:
  ReferenceFrame/RConn1 -- Solid/RConn1 -- F/RConn1

== system sm_import_stewart_platform/Stewart Platform/Imported Stewart Platform/ActuatorAssm2_2/CarrierAssm_1_RIGID/Hexagon_Socket_Button_Head_Screw_M3x6_6_RIGID ==
  ReferenceFrame : sm_lib/Frames and Transforms/Reference Frame
  Solid : sm_lib/Body Elements/File Solid  ExtGeomFileName=Hexagon_Socket_Button_Head_Screw_M3x6_Default_sldprt.STL  UnitType=Custom  ExtGeomFileUnits=cm  StepReaderType=HEX  ExportConvexHullGeometry=off  InertiaType=Custom  Mass=0.00056348185373580135  MassUnits=kg  CenterOfMass=[0.14356282026314221 8.1476592298985412e-06 5.8788316934839061e-08]  CenterOfMassUnits=cm  MomentsOfInertia=[1.3098988700385332e-05 3.5078394083955334e-05 3.5077439490752727e-05]  MomentsOfInertiaUnits=kg*cm^2  ProductsOfInertia=[-6.7519077190030419e-11 7.6873810692743504e-12 1.0654186206953444e-09]  ProductsOfInertiaUnits=kg*cm^2  BasedOnType=Density  Density=1000  DensityUnits=kg/(m^3)  DoExposeReferenceFrame=on  SerializedFrames=<Frames/>  GraphicType=FromGeometry  MarkerShape=Sphere  MarkerSize=10  MarkerSizeUnits=m  GraphicVisPropType=SimpleVisualProperties  GraphicDiffuseColor=[0.72282352941176464 0.72282352941176464 0.72282352941176464]  GraphicSpecularColor=[0.5 0.5 0.5 1.0]  GraphicAmbientColor=[0.15 0.15 0.15 1.0]  GraphicEmissiveColor=[0.0 0.0 0.0 1.0]  GraphicShininess=75  GraphicOpacity=1
  F : PMIOPort  Side=Left
  connections:
  ReferenceFrame/RConn1 -- Solid/RConn1 -- F/RConn1

== system sm_import_stewart_platform/Stewart Platform/Imported Stewart Platform/ActuatorAssm2_2/CarrierAssm_1_RIGID/Hexagon_Socket_Button_Head_Screw_M3x6_7_RIGID ==
  ReferenceFrame : sm_lib/Frames and Transforms/Reference Frame
  Solid : sm_lib/Body Elements/File Solid  ExtGeomFileName=Hexagon_Socket_Button_Head_Screw_M3x6_Default_sldprt.STL  UnitType=Custom  ExtGeomFileUnits=cm  StepReaderType=HEX  ExportConvexHullGeometry=off  InertiaType=Custom  Mass=0.00056348185373580135  MassUnits=kg  CenterOfMass=[0.14356282026314221 8.1476592298985412e-06 5.8788316934839061e-08]  CenterOfMassUnits=cm  MomentsOfInertia=[1.3098988700385332e-05 3.5078394083955334e-05 3.5077439490752727e-05]  MomentsOfInertiaUnits=kg*cm^2  ProductsOfInertia=[-6.7519077190030419e-11 7.6873810692743504e-12 1.0654186206953444e-09]  ProductsOfInertiaUnits=kg*cm^2  BasedOnType=Density  Density=1000  DensityUnits=kg/(m^3)  DoExposeReferenceFrame=on  SerializedFrames=<Frames/>  GraphicType=FromGeometry  MarkerShape=Sphere  MarkerSize=10  MarkerSizeUnits=m  GraphicVisPropType=SimpleVisualProperties  GraphicDiffuseColor=[0.72282352941176464 0.72282352941176464 0.72282352941176464]  GraphicSpecularColor=[0.5 0.5 0.5 1.0]  GraphicAmbientColor=[0.15 0.15 0.15 1.0]  GraphicEmissiveColor=[0.0 0.0 0.0 1.0]  GraphicShininess=75  GraphicOpacity=1
  F : PMIOPort  Side=Left
  connections:
  ReferenceFrame/RConn1 -- Solid/RConn1 -- F/RConn1

== system sm_import_stewart_platform/Stewart Platform/Imported Stewart Platform/ActuatorAssm2_2/CarrierAssm_1_RIGID/Hexagon_Socket_Button_Head_Screw_M3x6_8_RIGID ==
  ReferenceFrame : sm_lib/Frames and Transforms/Reference Frame
  Solid : sm_lib/Body Elements/File Solid  ExtGeomFileName=Hexagon_Socket_Button_Head_Screw_M3x6_Default_sldprt.STL  UnitType=Custom  ExtGeomFileUnits=cm  StepReaderType=HEX  ExportConvexHullGeometry=off  InertiaType=Custom  Mass=0.00056348185373580135  MassUnits=kg  CenterOfMass=[0.14356282026314221 8.1476592298985412e-06 5.8788316934839061e-08]  CenterOfMassUnits=cm  MomentsOfInertia=[1.3098988700385332e-05 3.5078394083955334e-05 3.5077439490752727e-05]  MomentsOfInertiaUnits=kg*cm^2  ProductsOfInertia=[-6.7519077190030419e-11 7.6873810692743504e-12 1.0654186206953444e-09]  ProductsOfInertiaUnits=kg*cm^2  BasedOnType=Density  Density=1000  DensityUnits=kg/(m^3)  DoExposeReferenceFrame=on  SerializedFrames=<Frames/>  GraphicType=FromGeometry  MarkerShape=Sphere  MarkerSize=10  MarkerSizeUnits=m  GraphicVisPropType=SimpleVisualProperties  GraphicDiffuseColor=[0.72282352941176464 0.72282352941176464 0.72282352941176464]  GraphicSpecularColor=[0.5 0.5 0.5 1.0]  GraphicAmbientColor=[0.15 0.15 0.15 1.0]  GraphicEmissiveColor=[0.0 0.0 0.0 1.0]  GraphicShininess=75  GraphicOpacity=1
  F : PMIOPort  Side=Left
  connections:
  ReferenceFrame/RConn1 -- Solid/RConn1 -- F/RConn1

== system sm_import_stewart_platform/Stewart Platform/Imported Stewart Platform/ActuatorAssm2_2/CarrierAssm_1_RIGID/Hexagon_Socket_Head_Cap_Screw_M3x5_1_RIGID ==
  ReferenceFrame : sm_lib/Frames and Transforms/Reference Frame
  Solid : sm_lib/Body Elements/File Solid  ExtGeomFileName=Hexagon_Socket_Head_Cap_Screw_M3x5_Default_sldprt.STL  UnitType=Custom  ExtGeomFileUnits=cm  StepReaderType=HEX  ExportConvexHullGeometry=off  InertiaType=Custom  Mass=0.00075563833672042757  MassUnits=kg  CenterOfMass=[-0.00070356125816108312 3.3976681789998727e-05 2.4288939549848704e-07]  CenterOfMassUnits=cm  MomentsOfInertia=[2.3283103549749918e-05 4.6860987295278262e-05 4.6851281632327237e-05]  MomentsOfInertiaUnits=kg*cm^2  ProductsOfInertia=[-6.6364273820729613e-10 4.0249100574764394e-11 5.6302615064034264e-09]  ProductsOfInertiaUnits=kg*cm^2  BasedOnType=Density  Density=1000  DensityUnits=kg/(m^3)  DoExposeReferenceFrame=on  SerializedFrames=<Frames/>  GraphicType=FromGeometry  MarkerShape=Sphere  MarkerSize=10  MarkerSizeUnits=m  GraphicVisPropType=SimpleVisualProperties  GraphicDiffuseColor=[0.72282352941176464 0.72282352941176464 0.72282352941176464]  GraphicSpecularColor=[0.5 0.5 0.5 1.0]  GraphicAmbientColor=[0.15 0.15 0.15 1.0]  GraphicEmissiveColor=[0.0 0.0 0.0 1.0]  GraphicShininess=75  GraphicOpacity=1
  F : PMIOPort  Side=Left
  connections:
  ReferenceFrame/RConn1 -- Solid/RConn1 -- F/RConn1

== system sm_import_stewart_platform/Stewart Platform/Imported Stewart Platform/ActuatorAssm2_2/CarrierAssm_1_RIGID/Hexagon_Socket_Head_Cap_Screw_M3x5_2_RIGID ==
  ReferenceFrame : sm_lib/Frames and Transforms/Reference Frame
  Solid : sm_lib/Body Elements/File Solid  ExtGeomFileName=Hexagon_Socket_Head_Cap_Screw_M3x5_Default_sldprt.STL  UnitType=Custom  ExtGeomFileUnits=cm  StepReaderType=HEX  ExportConvexHullGeometry=off  InertiaType=Custom  Mass=0.00075563833672042757  MassUnits=kg  CenterOfMass=[-0.00070356125816108312 3.3976681789998727e-05 2.4288939549848704e-07]  CenterOfMassUnits=cm  MomentsOfInertia=[2.3283103549749918e-05 4.6860987295278262e-05 4.6851281632327237e-05]  MomentsOfInertiaUnits=kg*cm^2  ProductsOfInertia=[-6.6364273820729613e-10 4.0249100574764394e-11 5.6302615064034264e-09]  ProductsOfInertiaUnits=kg*cm^2  BasedOnType=Density  Density=1000  DensityUnits=kg/(m^3)  DoExposeReferenceFrame=on  SerializedFrames=<Frames/>  GraphicType=FromGeometry  MarkerShape=Sphere  MarkerSize=10  MarkerSizeUnits=m  GraphicVisPropType=SimpleVisualProperties  GraphicDiffuseColor=[0.72282352941176464 0.72282352941176464 0.72282352941176464]  GraphicSpecularColor=[0.5 0.5 0.5 1.0]  GraphicAmbientColor=[0.15 0.15 0.15 1.0]  GraphicEmissiveColor=[0.0 0.0 0.0 1.0]  GraphicShininess=75  GraphicOpacity=1
  F : PMIOPort  Side=Left
  connections:
  ReferenceFrame/RConn1 -- Solid/RConn1 -- F/RConn1

== system sm_import_stewart_platform/Stewart Platform/Imported Stewart Platform/ActuatorAssm2_2/CarrierAssm_1_RIGID/Hexagon_Socket_Set_Screw_M3x3_1_RIGID ==
  ReferenceFrame : sm_lib/Frames and Transforms/Reference Frame
  Solid : sm_lib/Body Elements/File Solid  ExtGeomFileName=Hexagon_Socket_Set_Screw_M3x3_Default_sldprt.STL  UnitType=Custom  ExtGeomFileUnits=cm  StepReaderType=HEX  ExportConvexHullGeometry=off  InertiaType=Custom  Mass=0.00013414962639699338  MassUnits=kg  CenterOfMass=[0.14346797240988166 0 0]  CenterOfMassUnits=cm  MomentsOfInertia=[1.6122422751910497e-06 1.6862757603444589e-06 1.6862757577761036e-06]  MomentsOfInertiaUnits=kg*cm^2  ProductsOfInertia=[0 0 0]  ProductsOfInertiaUnits=kg*cm^2  BasedOnType=Density  Density=1000  DensityUnits=kg/(m^3)  DoExposeReferenceFrame=on  SerializedFrames=<Frames/>  GraphicType=FromGeometry  MarkerShape=Sphere  MarkerSize=10  MarkerSizeUnits=m  GraphicVisPropType=SimpleVisualProperties  GraphicDiffuseColor=[0.72282352941176464 0.72282352941176464 0.72282352941176464]  GraphicSpecularColor=[0.5 0.5 0.5 1.0]  GraphicAmbientColor=[0.15 0.15 0.15 1.0]  GraphicEmissiveColor=[0.0 0.0 0.0 1.0]  GraphicShininess=75  GraphicOpacity=1
  F : PMIOPort  Side=Left
  connections:
  ReferenceFrame/RConn1 -- Solid/RConn1 -- F/RConn1

== system sm_import_stewart_platform/Stewart Platform/Imported Stewart Platform/ActuatorAssm2_2/CarrierAssm_1_RIGID/Hexagon_Socket_Set_Screw_M3x3_2_RIGID ==
  ReferenceFrame : sm_lib/Frames and Transforms/Reference Frame
  Solid : sm_lib/Body Elements/File Solid  ExtGeomFileName=Hexagon_Socket_Set_Screw_M3x3_Default_sldprt.STL  UnitType=Custom  ExtGeomFileUnits=cm  StepReaderType=HEX  ExportConvexHullGeometry=off  InertiaType=Custom  Mass=0.00013414962639699338  MassUnits=kg  CenterOfMass=[0.14346797240988166 0 0]  CenterOfMassUnits=cm  MomentsOfInertia=[1.6122422751910497e-06 1.6862757603444589e-06 1.6862757577761036e-06]  MomentsOfInertiaUnits=kg*cm^2  ProductsOfInertia=[0 0 0]  ProductsOfInertiaUnits=kg*cm^2  BasedOnType=Density  Density=1000  DensityUnits=kg/(m^3)  DoExposeReferenceFrame=on  SerializedFrames=<Frames/>  GraphicType=FromGeometry  MarkerShape=Sphere  MarkerSize=10  MarkerSizeUnits=m  GraphicVisPropType=SimpleVisualProperties  GraphicDiffuseColor=[0.72282352941176464 0.72282352941176464 0.72282352941176464]  GraphicSpecularColor=[0.5 0.5 0.5 1.0]  GraphicAmbientColor=[0.15 0.15 0.15 1.0]  GraphicEmissiveColor=[0.0 0.0 0.0 1.0]  GraphicShininess=75  GraphicOpacity=1
  F : PMIOPort  Side=Left
  connections:
  ReferenceFrame/RConn1 -- Solid/RConn1 -- F/RConn1

== system sm_import_stewart_platform/Stewart Platform/Imported Stewart Platform/ActuatorAssm2_2/CarrierAssm_1_RIGID/Hexagon_Socket_Set_Screw_M3x3_3_RIGID ==
  ReferenceFrame : sm_lib/Frames and Transforms/Reference Frame
  Solid : sm_lib/Body Elements/File Solid  ExtGeomFileName=Hexagon_Socket_Set_Screw_M3x3_Default_sldprt.STL  UnitType=Custom  ExtGeomFileUnits=cm  StepReaderType=HEX  ExportConvexHullGeometry=off  InertiaType=Custom  Mass=0.00013414962639699338  MassUnits=kg  CenterOfMass=[0.14346797240988166 0 0]  CenterOfMassUnits=cm  MomentsOfInertia=[1.6122422751910497e-06 1.6862757603444589e-06 1.6862757577761036e-06]  MomentsOfInertiaUnits=kg*cm^2  ProductsOfInertia=[0 0 0]  ProductsOfInertiaUnits=kg*cm^2  BasedOnType=Density  Density=1000  DensityUnits=kg/(m^3)  DoExposeReferenceFrame=on  SerializedFrames=<Frames/>  GraphicType=FromGeometry  MarkerShape=Sphere  MarkerSize=10  MarkerSizeUnits=m  GraphicVisPropType=SimpleVisualProperties  GraphicDiffuseColor=[0.72282352941176464 0.72282352941176464 0.72282352941176464]  GraphicSpecularColor=[0.5 0.5 0.5 1.0]  GraphicAmbientColor=[0.15 0.15 0.15 1.0]  GraphicEmissiveColor=[0.0 0.0 0.0 1.0]  GraphicShininess=75  GraphicOpacity=1
  F : PMIOPort  Side=Left
  connections:
  ReferenceFrame/RConn1 -- Solid/RConn1 -- F/RConn1

== system sm_import_stewart_platform/Stewart Platform/Imported Stewart Platform/ActuatorAssm2_2/CarrierAssm_1_RIGID/Hexagon_Socket_Set_Screw_M3x3_4_RIGID ==
  ReferenceFrame : sm_lib/Frames and Transforms/Reference Frame
  Solid : sm_lib/Body Elements/File Solid  ExtGeomFileName=Hexagon_Socket_Set_Screw_M3x3_Default_sldprt.STL  UnitType=Custom  ExtGeomFileUnits=cm  StepReaderType=HEX  ExportConvexHullGeometry=off  InertiaType=Custom  Mass=0.00013414962639699338  MassUnits=kg  CenterOfMass=[0.14346797240988166 0 0]  CenterOfMassUnits=cm  MomentsOfInertia=[1.6122422751910497e-06 1.6862757603444589e-06 1.6862757577761036e-06]  MomentsOfInertiaUnits=kg*cm^2  ProductsOfInertia=[0 0 0]  ProductsOfInertiaUnits=kg*cm^2  BasedOnType=Density  Density=1000  DensityUnits=kg/(m^3)  DoExposeReferenceFrame=on  SerializedFrames=<Frames/>  GraphicType=FromGeometry  MarkerShape=Sphere  MarkerSize=10  MarkerSizeUnits=m  GraphicVisPropType=SimpleVisualProperties  GraphicDiffuseColor=[0.72282352941176464 0.72282352941176464 0.72282352941176464]  GraphicSpecularColor=[0.5 0.5 0.5 1.0]  GraphicAmbientColor=[0.15 0.15 0.15 1.0]  GraphicEmissiveColor=[0.0 0.0 0.0 1.0]  GraphicShininess=75  GraphicOpacity=1
  F : PMIOPort  Side=Left
  connections:
  ReferenceFrame/RConn1 -- Solid/RConn1 -- F/RConn1

== system sm_import_stewart_platform/Stewart Platform/Imported Stewart Platform/ActuatorAssm2_2/CarrierAssm_1_RIGID/Hexagon_Socket_Set_Screw_M3x3_5_RIGID ==
  ReferenceFrame : sm_lib/Frames and Transforms/Reference Frame
  Solid : sm_lib/Body Elements/File Solid  ExtGeomFileName=Hexagon_Socket_Set_Screw_M3x3_Default_sldprt.STL  UnitType=Custom  ExtGeomFileUnits=cm  StepReaderType=HEX  ExportConvexHullGeometry=off  InertiaType=Custom  Mass=0.00013414962639699338  MassUnits=kg  CenterOfMass=[0.14346797240988166 0 0]  CenterOfMassUnits=cm  MomentsOfInertia=[1.6122422751910497e-06 1.6862757603444589e-06 1.6862757577761036e-06]  MomentsOfInertiaUnits=kg*cm^2  ProductsOfInertia=[0 0 0]  ProductsOfInertiaUnits=kg*cm^2  BasedOnType=Density  Density=1000  DensityUnits=kg/(m^3)  DoExposeReferenceFrame=on  SerializedFrames=<Frames/>  GraphicType=FromGeometry  MarkerShape=Sphere  MarkerSize=10  MarkerSizeUnits=m  GraphicVisPropType=SimpleVisualProperties  GraphicDiffuseColor=[0.72282352941176464 0.72282352941176464 0.72282352941176464]  GraphicSpecularColor=[0.5 0.5 0.5 1.0]  GraphicAmbientColor=[0.15 0.15 0.15 1.0]  GraphicEmissiveColor=[0.0 0.0 0.0 1.0]  GraphicShininess=75  GraphicOpacity=1
  F : PMIOPort  Side=Left
  connections:
  ReferenceFrame/RConn1 -- Solid/RConn1 -- F/RConn1
